simulink model "balanceBotNonlin"  (R2019b)
settings: Solver=VariableStepAuto  StartTime=0.0  StopTime=10.0  RelTol=1e-3
values from neighbouring files (symbols this model uses):
  A = [0      1              0           0 ... (first row only)    [BalanceBotMBC.m]    (also in BalanceBotPetruska.m = W*Ap*inv(W); obs_ctrl_example_script.m = [0 1 0; 0 0 1; -15 -7 -3;])
  B = [     0 ... (first row only)    [BalanceBotMBC.m]    (also in BalanceBotPetruska.m = W*Bp; obs_ctrl_example_script.m = [0;0;23])
  C = [1 0 0 0 ... (first row only)    [BalanceBotMBC.m]    (also in BalanceBotPetruska.m = [ C_row1; obs_ctrl_example_script.m = [1 0 0])
  D = [0 ... (first row only)    [BalanceBotMBC.m]    (also in BalanceBotPetruska.m = [ D_row1; obs_ctrl_example_script.m = 0)
  Kd = place(Ad,Bd,des_p_ctrl_d)    [BalanceBotMBC.m]    (also in obs_ctrl_example_script.m = place(Ad,Bd,cl_poles_disc))
  Ld = place(Ad',(Cd*Ad)',des_p_obs_d)'    [BalanceBotMBC.m]    (also in obs_ctrl_example_script.m = place(Ad',(C*Ad)',obs_poles)')
settings Model: EnablePacing=on  Creator=Matthew  LastModifiedBy=Matthew

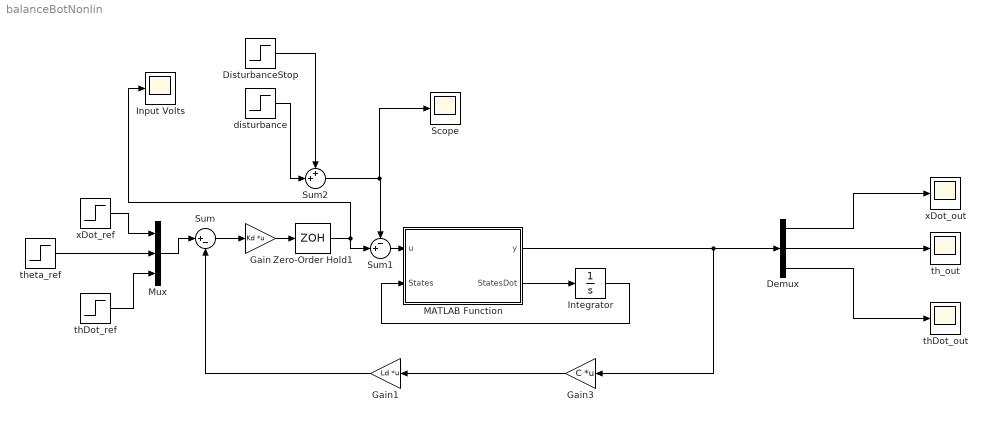
== system balanceBotNonlin ==
  Demux : Demux  Outputs=3
  DisturbanceStop : Step  Time=1.2  After=-.1  SampleTime=0
  Gain : Gain  Gain=Kd  Multiplication=Matrix(K*u)
  Gain1 : Gain  Gain=Ld  Multiplication=Matrix(K*u)
  Gain3 : Gain  Gain=C  Multiplication=Matrix(K*u)
  Input Volts : Scope
  Integrator : Integrator  InitialCondition=[0;pi;0]
  MATLAB Function : MATLAB Function  TreatAsAtomicUnit=on
  Mux : Mux  Inputs=3
  Scope : Scope
  Sum : Sum  Inputs=|+-
  Sum1 : Sum  Inputs=-+|
  Sum2 : Sum  Inputs=++|
  Zero-Order Hold1 : ZeroOrderHold  SampleTime=.001
  disturbance : Step  After=.1  SampleTime=0
  thDot_out : Scope
  thDot_ref : Step  After=0  SampleTime=0
  th_out : Scope
  theta_ref : Step  Before=pi  After=pi  SampleTime=0
  xDot_out : Scope
  xDot_ref : Step  After=0  SampleTime=0
  wires:
  xDot_ref/1 -> Mux/1
  theta_ref/1 -> Mux/2
  Mux/1 -> Sum/1
  Sum/1 -> Gain/1
  Gain1/1 -> Sum/2
  Demux/1 -> xDot_out/1
  Demux/2 -> th_out/1
  thDot_ref/1 -> Mux/3
  Sum1/1 -> MATLAB Function/1(u)
  disturbance/1 -> Sum2/2
  DisturbanceStop/1 -> Sum2/1
  Demux/3 -> thDot_out/1
  MATLAB Function/1(y) -> Gain3/1, Demux/1
  MATLAB Function/2(StatesDot) -> Integrator/1
  Integrator/1 -> MATLAB Function/2(States)
  Gain3/1 -> Gain1/1
  Gain/1 -> Zero-Order Hold1/1
  Zero-Order Hold1/1 -> Sum1/2, Input Volts/1
  Sum2/1 -> Scope/1, Sum1/1

== matlab function balanceBotNonlin/MATLAB Function ==
  data: u input; y output; States input; StatesDot output; A parameter; B parameter; C parameter; D parameter
function [y, StatesDot] = fcn(u,States,A, B, C, D)
    
    StatesDot = A*States + B*u;
    y = States;
